simulink model "x1"  (R2019b)
settings: Solver=VariableStepAuto  StartTime=0.0  StopTime=10.0  RelTol=1e-3
undefined symbols (not defined in the file): ini_x1, ini_x1_d, r1
settings Model: Creator=mic-ciciolla  LastModifiedBy=mic-ciciolla

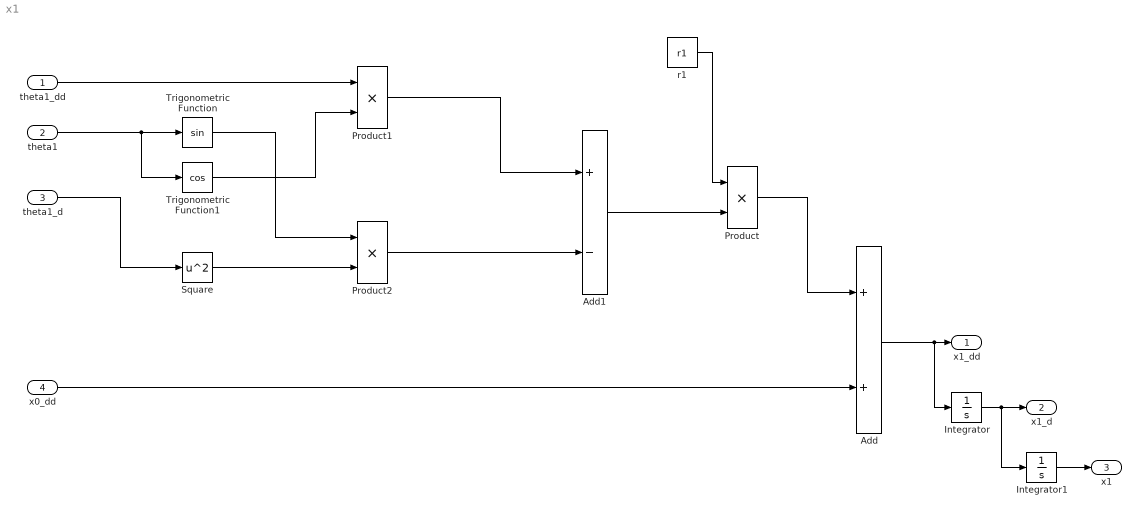
== system x1 ==
  "theta1_dd " : Inport
  theta1 : Inport  Port=2
  theta1_d : Inport  Port=3
  x0_dd : Inport  Port=4
  Add : Sum
  Add1 : Sum  Inputs=+-
  Integrator : Integrator  InitialCondition=ini_x1_d
  Integrator1 : Integrator  InitialCondition=ini_x1
  Product : Product
  Product1 : Product
  Product2 : Product
  Square : Math  Operator=square  SignedPower=off  SaturateOnIntegerOverflow=on
  Trigonometric Function : Trigonometry
  Trigonometric Function1 : Trigonometry  Operator=cos
  r1 : Constant  Value=r1
  x1_dd : Outport
  x1_d : Outport  Port=2
  x1 : Outport  Port=3
  wires:
  Add1/1 -> Product/2
  Add/1 -> Integrator/1, x1_dd/1
  Product/1 -> Add/1
  Square/1 -> Product2/2
  r1/1 -> Product/1
  Integrator1/1 -> x1/1
  theta1/1 -> Trigonometric Function1/1, Trigonometric Function/1
  theta1_d/1 -> Square/1
  x0_dd/1 -> Add/2
  Product1/1 -> Add1/1
  "theta1_dd "/1 -> Product1/1
  Integrator/1 -> Integrator1/1, x1_d/1
  Product2/1 -> Add1/2
  Trigonometric Function1/1 -> Product1/2
  Trigonometric Function/1 -> Product2/1
